simulink model "Test"  (R2021b)
settings: Solver=VariableStepAuto  StartTime=0.0  StopTime=600.0  RelTol=1e-3
libraries: sharedtransform x1
settings Model: Creator=aakas  LastModifiedBy=aakas

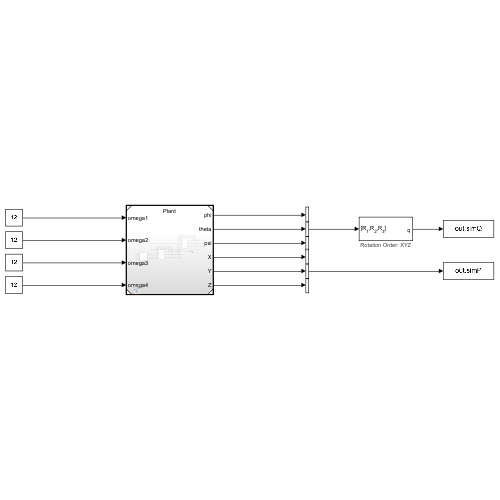
[thumbnail: Simulink's stored preview of the top-level diagram]
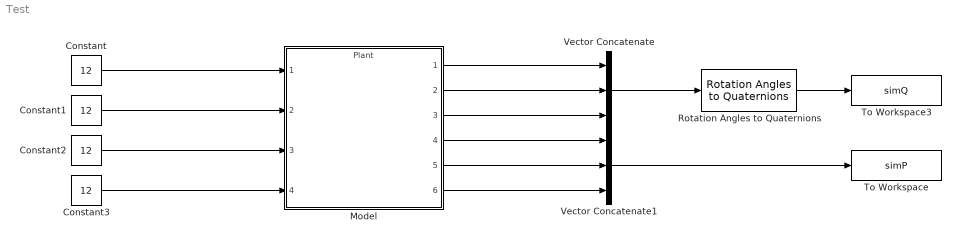
== system Test ==
  Constant{,1..3} (4 alike) : Constant  Value=12  SampleTime=0.001
  Model : ModelReference  ModelNameDialog=Plant.slx  SimulationMode=Normal  ModelReferenceVersion=1.13
  Rotation Angles to Quaternions : sharedtransform/Rotation Angles to Quaternions  rotationOrder=XYZ  aMode=aMode
      settings: SourceProductBaseCode=AE,PW,DR,MT,UV,VE
  To Workspace : ToWorkspace  VariableName=simP  SampleTime=-1
  To Workspace3 : ToWorkspace  VariableName=simQ  SampleTime=-1
  Vector Concatenate : Concatenate  NumInputs=3
  Vector Concatenate1 : Concatenate  NumInputs=3
  wires:
  Model/1 -> Vector Concatenate/1
  Model/2 -> Vector Concatenate/2
  Model/3 -> Vector Concatenate/3
  Model/4 -> Vector Concatenate1/1
  Model/5 -> Vector Concatenate1/2
  Model/6 -> Vector Concatenate1/3
  Vector Concatenate/1 -> Rotation Angles to Quaternions/1
  Rotation Angles to Quaternions/1 -> To Workspace3/1
  Vector Concatenate1/1 -> To Workspace/1
  Constant/1 -> Model/1
  Constant1/1 -> Model/2
  Constant2/1 -> Model/3
  Constant3/1 -> Model/4
